simulink model "PD_funcional2018"  (R2023a)
settings: Solver=ode4  StartTime=0.0  StopTime=5  FixedStep=1e-4  RelTol=1e-3
StopFcn:
  | out = evalin('base','out');
  | animar_pendulo(out,30)
model workspace (MAT data in the model file):
  sample_time = 0.001
  sat_limit = 10
libraries: eeGeneralControl x1

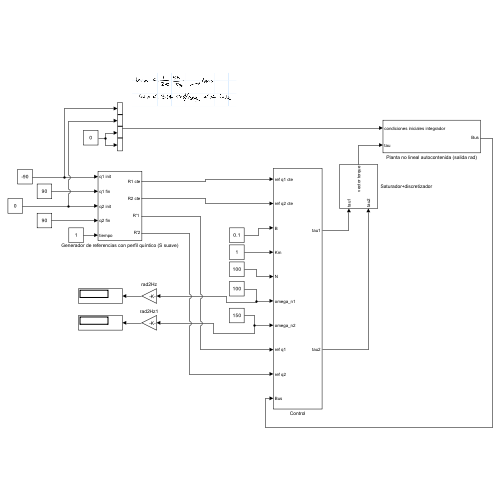
[thumbnail: Simulink's stored preview of the top-level diagram]
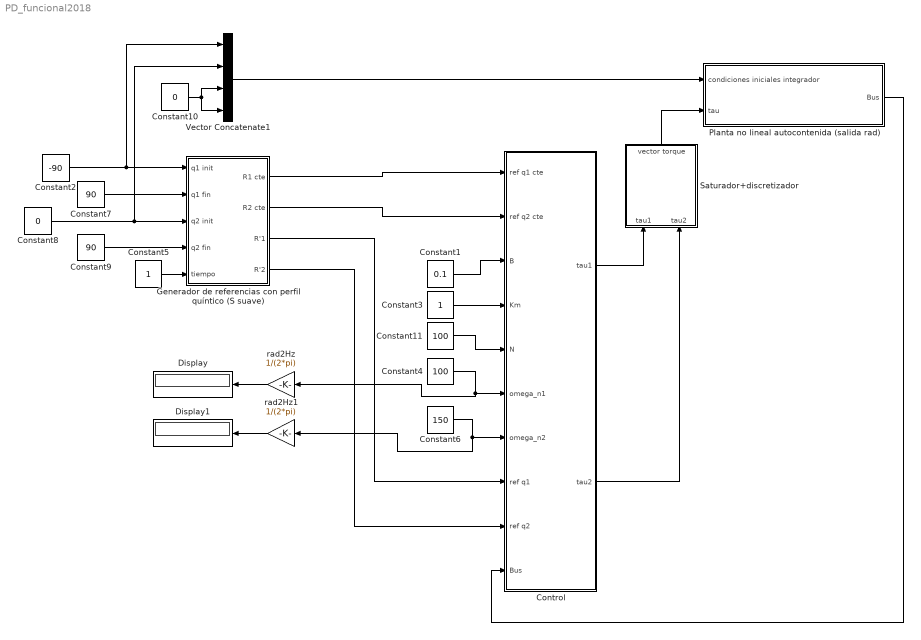
== system PD_funcional2018 ==
  Constant1 : Constant  Value=0.1
  Constant10 : Constant  Value=0
  Constant11 : Constant  Value=100
  Constant2 : Constant  Value=-90
  Constant3 : Constant
  Constant4 : Constant  Value=100
  Constant5 : Constant
  Constant6 : Constant  Value=150
  Constant7 : Constant  Value=90
  Constant8 : Constant  Value=0
  Constant9 : Constant  Value=90
  Control : Subsystem
  Display : Display
  Display1 : Display
  Generador de referencias con perfil quíntico (S suave) : Subsystem
  Planta no lineal autocontenida (salida rad) : Subsystem
  Saturador+discretizador : Subsystem
  Vector Concatenate1 : Concatenate  NumInputs=4
  rad2Hz : Gain  Gain=1/(2*pi)
  rad2Hz1 : Gain  Gain=1/(2*pi)
  wires:
  Constant2/1 -> Generador de referencias con perfil quíntico (S suave)/1(q1 init), Vector Concatenate1/1
  Constant7/1 -> Generador de referencias con perfil quíntico (S suave)/2(q1 fin)
  Constant8/1 -> Vector Concatenate1/2, Generador de referencias con perfil quíntico (S suave)/3(q2 init)
  Constant9/1 -> Generador de referencias con perfil quíntico (S suave)/4(q2 fin)
  Constant5/1 -> Generador de referencias con perfil quíntico (S suave)/5(tiempo)
  Saturador+discretizador/1(vector torque) -> Planta no lineal autocontenida (salida rad)/2(tau)
  Constant10/1 -> Vector Concatenate1/3, Vector Concatenate1/4
  Vector Concatenate1/1 -> Planta no lineal autocontenida (salida rad)/1(condiciones iniciales integrador)
  Generador de referencias con perfil quíntico (S suave)/1(R1 cte) -> Control/1(ref q1 cte)
  Generador de referencias con perfil quíntico (S suave)/2(R2 cte) -> Control/2(ref q2 cte)
  Constant1/1 -> Control/3(B)
  Constant3/1 -> Control/4(Km)
  Constant4/1 -> rad2Hz/1, Control/6(omega_n1)
  Constant6/1 -> rad2Hz1/1, Control/7(omega_n2)
  Control/1(tau1) -> Saturador+discretizador/1(tau1)
  Planta no lineal autocontenida (salida rad)/1(Bus) -> Control/10(Bus)
  Generador de referencias con perfil quíntico (S suave)/3("R'1 ") -> Control/8(ref q1)
  Generador de referencias con perfil quíntico (S suave)/4(R'2) -> Control/9(ref q2)
  rad2Hz/1 -> Display/1
  rad2Hz1/1 -> Display1/1
  Control/2(tau2) -> Saturador+discretizador/2(tau2)
  Constant11/1 -> Control/5(N)

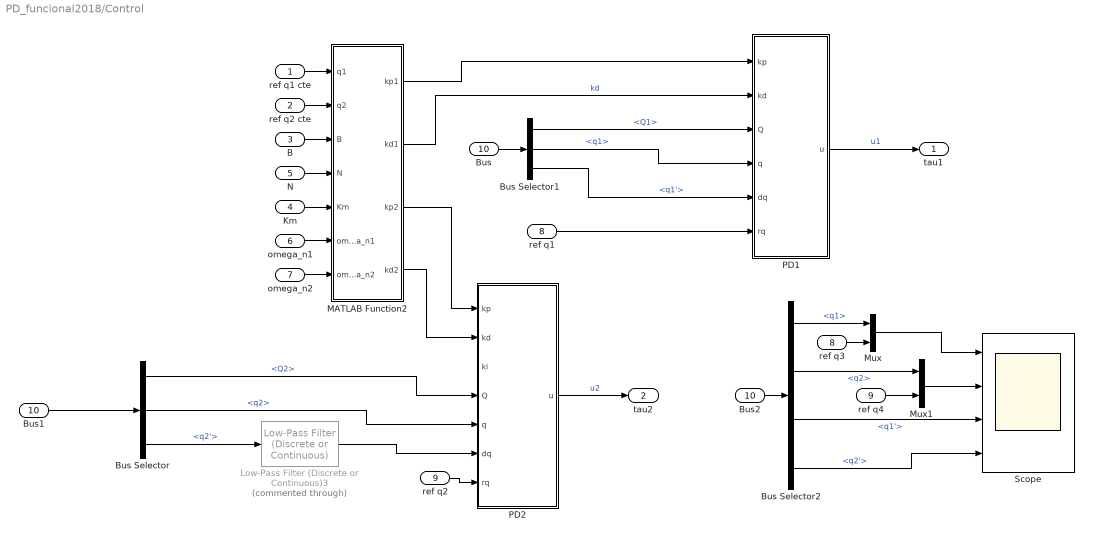
== system PD_funcional2018/Control ==
  ref q1 cte : Inport
  ref q2 cte : Inport  Port=2
  B : Inport  Port=3
  Km : Inport  Port=4
  N : Inport  Port=5
  omega_n1 : Inport  Port=6
  omega_n2 : Inport  Port=7
  ref q1 : Inport  Port=8
  ref q2 : Inport  Port=9
  Bus : Inport  Port=10
  Bus Selector : BusSelector  OutputSignals=Q2,q2,q2'
  Bus Selector1 : BusSelector  OutputSignals=Q1,q1,q1'
  Bus Selector2 : BusSelector  OutputSignals=q1,q2,q1',q2'
  Bus1 : InportShadow  Port=10
  Bus2 : InportShadow  Port=10
  Low-Pass Filter (Discrete or Continuous)3 : eeGeneralControl/Low-Pass Filter (Discrete or Continuous)  Commented=through  K=1  T=1/30  B=inf  A=-inf  init_option=Inherited from block input  x0=0  Ts=-1
  MATLAB Function2 : MATLAB Function  TreatAsAtomicUnit=on
  Mux : Mux  Inputs=2
  Mux1 : Mux  Inputs=2
  PD1 : MATLAB Function  TreatAsAtomicUnit=on
  PD2 : MATLAB Function  TreatAsAtomicUnit=on
  Scope : Scope  NumInputPorts=4
  ref q3 : InportShadow  Port=8
  ref q4 : InportShadow  Port=9
  tau1 : Outport
  tau2 : Outport  Port=2
  wires:
  ref q1 cte/1 -> MATLAB Function2/1(q1)
  ref q2 cte/1 -> MATLAB Function2/2(q2)
  B/1 -> MATLAB Function2/3(B)
  omega_n2/1 -> MATLAB Function2/7(omega_n2)
  omega_n1/1 -> MATLAB Function2/6(omega_n1)
  PD1/1(u) -> tau1/1  "u1"
  PD2/1(u) -> tau2/1  "u2"
  ref q1/1 -> PD1/6(rq)
  ref q2/1 -> PD2/7(rq)
  MATLAB Function2/1(kp1) -> PD1/1(kp)
  MATLAB Function2/3(kp2) -> PD2/1(kp)
  MATLAB Function2/2(kd1) -> PD1/2(kd)  "kd"
  MATLAB Function2/4(kd2) -> PD2/2(kd)
  Bus1/1 -> Bus Selector/1
  Bus/1 -> Bus Selector1/1
  Bus Selector1/1 -> PD1/3(Q)  "<Q1>"
  Bus Selector1/2 -> PD1/4(q)  "<q1>"
  Bus Selector1/3 -> PD1/5(dq)  "<q1'>"
  Bus Selector/1 -> PD2/4(Q)  "<Q2>"
  Bus Selector/3 -> Low-Pass Filter (Discrete or Continuous)3/1  "<q2'>"
  Mux/1 -> Scope/1
  Mux1/1 -> Scope/2
  Bus2/1 -> Bus Selector2/1
  Bus Selector2/1 -> Mux/1  "<q1>"
  Bus Selector2/2 -> Mux1/1  "<q2>"
  Bus Selector2/3 -> Scope/3  "<q1'>"
  Bus Selector2/4 -> Scope/4  "<q2'>"
  ref q3/1 -> Mux/2
  ref q4/1 -> Mux1/2
  Bus Selector/2 -> PD2/5(q)  "<q2>"
  Low-Pass Filter (Discrete or Continuous)3/1 -> PD2/6(dq)
  Km/1 -> MATLAB Function2/5(Km)
  N/1 -> MATLAB Function2/4(N)

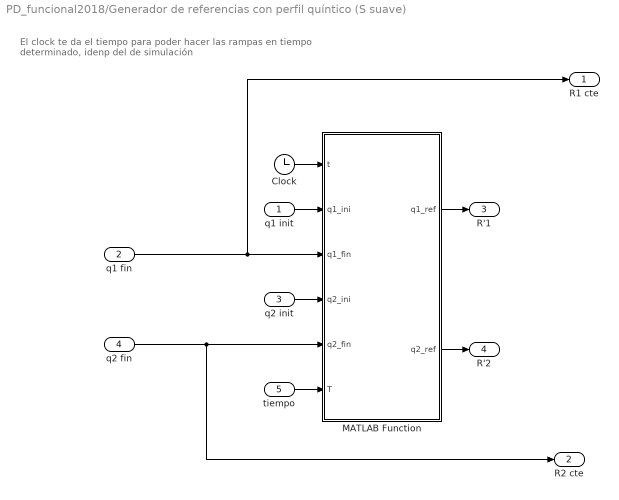
== system PD_funcional2018/Generador de referencias con perfil quíntico (S suave) ==
  note: El clock te da el tiempo para poder hacer las rampas en tiempo determinado, idenp del de simulación
  q1 init : Inport
  q1 fin : Inport  Port=2
  q2 init : Inport  Port=3
  q2 fin : Inport  Port=4
  tiempo : Inport  Port=5
  Clock : Clock
  MATLAB Function : MATLAB Function  TreatAsAtomicUnit=on
  R1 cte : Outport
  R2 cte : Outport  Port=2
  "R'1 " : Outport  Port=3
  R'2 : Outport  Port=4
  wires:
  q1 fin/1 -> R1 cte/1, MATLAB Function/3(q1_fin)
  q2 fin/1 -> R2 cte/1, MATLAB Function/5(q2_fin)
  q1 init/1 -> MATLAB Function/2(q1_ini)
  q2 init/1 -> MATLAB Function/4(q2_ini)
  MATLAB Function/1(q1_ref) -> "R'1 "/1
  MATLAB Function/2(q2_ref) -> R'2/1
  tiempo/1 -> MATLAB Function/6(T)
  Clock/1 -> MATLAB Function/1(t)

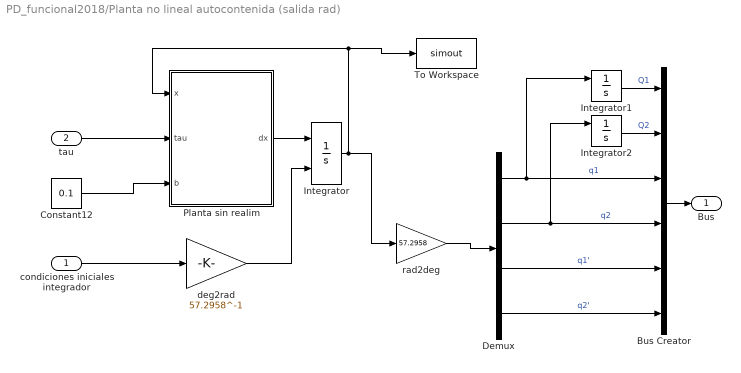
== system PD_funcional2018/Planta no lineal autocontenida (salida rad) ==
  condiciones iniciales integrador : Inport
  tau : Inport  Port=2
  Bus Creator : BusCreator  Inputs=6
  Constant12 : Constant  Value=0.1
  Demux : Demux
  Integrator : Integrator  InitialConditionSource=external
  Integrator1 : Integrator  InitialConditionSource=external
  Integrator2 : Integrator  InitialConditionSource=external
  Planta sin realim : MATLAB Function  TreatAsAtomicUnit=on
  To Workspace : ToWorkspace  VariableName=simout  SaveFormat=Structure With Time  SampleTime=-1
  deg2rad : Gain  Gain=57.2958^-1
  rad2deg : Gain  Gain=57.2958
  Bus : Outport
  wires:
  tau/1 -> Planta sin realim/2(tau)
  Constant12/1 -> Planta sin realim/3(b)
  Integrator/1 -> Planta sin realim/1(x), To Workspace/1, rad2deg/1
  condiciones iniciales integrador/1 -> deg2rad/1
  Planta sin realim/1(dx) -> Integrator/1
  deg2rad/1 -> Integrator/2
  rad2deg/1 -> Demux/1
  Demux/1 -> Integrator1/1, Bus Creator/3  "q1"
  Demux/2 -> Integrator2/1, Bus Creator/4  "q2"
  Demux/3 -> Bus Creator/5  "q1'"
  Demux/4 -> Bus Creator/6  "q2'"
  Integrator1/1 -> Bus Creator/1  "Q1"
  Integrator2/1 -> Bus Creator/2  "Q2"
  Bus Creator/1 -> Bus/1

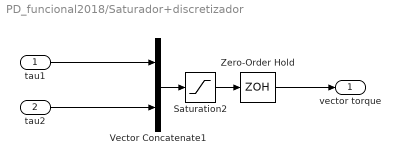
== system PD_funcional2018/Saturador+discretizador ==
  tau1 : Inport
  tau2 : Inport  Port=2
  Saturation2 : Saturate  UpperLimit=sat_limit  LowerLimit=-sat_limit
  Vector Concatenate1 : Concatenate
  Zero-Order Hold : ZeroOrderHold  SampleTime=sample_time
  vector torque : Outport
  wires:
  tau2/1 -> Vector Concatenate1/2
  tau1/1 -> Vector Concatenate1/1
  Saturation2/1 -> Zero-Order Hold/1
  Vector Concatenate1/1 -> Saturation2/1
  Zero-Order Hold/1 -> vector torque/1

== matlab function PD_funcional2018/Control/PD1 ==
function u  = PD(kp,kd,Q,q,dq,rq)
error = rq - q;
u = kp*error - kd * dq;
end

== matlab function PD_funcional2018/Planta no lineal autocontenida (salida rad)/Planta sin realim ==
function dx = modelo_estado(x, tau, b)
% MODELO_ESTADO  Bloque MATLAB Function para Simulink — formulación SS no lineal.
% Devuelve la derivada del vector de estado completo.
%
% Entradas:
%   x   = [q1; q2; dq1; dq2]  (4x1)
%   tau = [tau1; tau2]         (2x1)
%
% Salida:
%   dx  = [dq1; dq2; ddq1; ddq2]  (4x1)
%
% Conectar: un bloque Integrator vectorial (IC = x0, 4 estados)
%           con retroalimentación completa de x.

q1  = x(1);
q2  = x(2);
dq1 = x(3);
dq2 = x(4);

[ddq1, ddq2] = dinamica_fcn(q1, q2, dq1, dq2, tau(1), tau(2),b);

dx = [dq1; dq2; ddq1; ddq2];
end


function [ddq1, ddq2] = dinamica_fcn(q1, q2, dq1, dq2, tau1, tau2,b)
% DINAMICA_FCN  Bloque MATLAB Function para Simulink.
% Calcula las aceleraciones articulares del doble péndulo invertido.
% Modelo: tau = M(q)*ddq + H(q,dq) + G(q)  =>  ddq = M^-1*(tau - H - G)
%
% Notación: c1=cos(q1), s1=sin(q1), c12=cos(q1+q2), s12=sin(q1+q2), c2=cos(q2)

% --- Parámetros (hardcoded para el bloque) ---
a1    = 0.2;
a2    = 0.2;
m1    = 1.5;
m2    = 1.0;
Ig1zz = 1e-3;
Ig2zz = 1e-4;
xg1   = -a1/2;   % = -0.1
yg1   = 0;
xg2   = -a2/2;   % = -0.1
yg2   = 0;
grav  = 9.81;

% --- Trigonometría ---
c1  = cos(q1);
s1  = sin(q1);
c2  = cos(q2);
s2  = sin(q2);
c12 = cos(q1 + q2);
s12 = sin(q1 + q2);

% --- Matriz de inercia M (ec. 27-30 de la memoria) ---
% I0izz = Igizz + (xgi^2 + ygi^2)*mi  [Steiner, para la terna del eslabón]
I01zz = Ig1zz + (xg1^2 + yg1^2)*m1;   % = 0.016 Kg·m²
I02zz = Ig2zz + (xg2^2 + yg2^2)*m2;   % = 0.0101 Kg·m²  (aprox, yg2=0)

m22 = I02zz + 2*a2*xg2*m2 + a2^2*m2;
m12 = m22 + a1*((a2 + xg2)*c2 - yg2*s2)*m2;
m11 = I01zz + 2*a1*xg1*m1 + a1^2*(m1 + m2) + 2*m12 - m22;

M = [m11, m12; m12, m22];

% --- Vector H — Coriolis y centrífugo (ec. 33) ---
dm12_dq2 = -a1*((a2 + xg2)*s2 + yg2*c2)*m2;

H1 = dm12_dq2 * (2*dq1*dq2 + dq2^2);
H2 = -dm12_dq2 * dq1^2;

H = [H1; H2];

% --- Vector G — gravedad (ec. 36, 40) ---
% g^0 = [0, -9.81, 0]^t  (montado en la pared, gravedad en -Y de frame 0)
g2 = m2*grav*((xg2 + a2)*c12 - yg2*s12);
g1 = m1*grav*((xg1 + a1)*c1 - yg1*s1) + m2*grav*a1*c1 + g2;

G = [g1; g2];

B = [dq1; dq2] * b; % fricción simplificada

% --- Ecuación de movimiento ---
tau = [tau1; tau2];
ddq = M \ (tau - H - G - B); % no está dividiendo, esta resolviendo con división de M a izquierda
% B es fricción 

ddq1 = ddq(1);
ddq2 = ddq(2);
end

== matlab function PD_funcional2018/Control/MATLAB Function2 ==
function [kp1,kd1,kp2,kd2] = coefs_PD(q1,q2,B,N,Km,omega_n1,omega_n2)
%e error
[Jef1,Jef2] = Matriz_M_eq(q1,q2);

kp1 = (omega_n1^2)*Jef1 / (N*Km);
kd1 = (2 * sqrt(N*Km*kp1*Jef1)- B)/(N*Km); 

kp2 = (omega_n2^2)*Jef2 / (N*Km);
kd2 = (2 * sqrt(N*Km*kp2*Jef2)- B)/(N*Km); 

end

function [m11,m22] = Matriz_M_eq(q1, q2)
% DINAMICA_FCN  Bloque MATLAB Function para Simulink.
% Calcula las aceleraciones articulares del doble péndulo invertido.
% Modelo: tau = M(q)*ddq + H(q,dq) + G(q)  =>  ddq = M^-1*(tau - H - G)
%
% Notación: c1=cos(q1), s1=sin(q1), c12=cos(q1+q2), s12=sin(q1+q2), c2=cos(q2)

% --- Parámetros (hardcoded para el bloque) ---
a1    = 0.2;
a2    = 0.2;
m1    = 1.5;
m2    = 1.0;
Ig1zz = 1e-3;
Ig2zz = 1e-4;
xg1   = -a1/2;   % = -0.1
yg1   = 0;
xg2   = -a2/2;   % = -0.1
yg2   = 0;
grav  = 9.81;

q1 = deg2rad(q1);
q2 = deg2rad(q2);

% --- Trigonometría ---
c1  = cos(q1);
s1  = sin(q1);
c2  = cos(q2);
s2  = sin(q2);
c12 = cos(q1 + q2);
s12 = sin(q1 + q2);

% --- Matriz de inercia M (ec. 27-30 de la memoria) ---
% I0izz = Igizz + (xgi^2 + ygi^2)*mi  [Steiner, para la terna del eslabón]
I01zz = Ig1zz + (xg1^2 + yg1^2)*m1;   % = 0.016 Kg·m²
I02zz = Ig2zz + (xg2^2 + yg2^2)*m2;   % = 0.0101 Kg·m²  (aprox, yg2=0)

m22 = I02zz + 2*a2*xg2*m2 + a2^2*m2;
m12 = m22 + a1*((a2 + xg2)*c2 - yg2*s2)*m2;
m11 = I01zz + 2*a1*xg1*m1 + a1^2*(m1 + m2) + 2*m12 - m22;

M = [m11, m12; m12, m22];

m11=m11;
m12=m12;
m21=m12;
m22=m22;
end

== matlab function PD_funcional2018/Control/PD2 ==
function u  = PD(kp,kd,ki,Q,q,dq,rq)
error = rq - q;
u = kp*error - kd * dq;
end

== matlab function PD_funcional2018/Generador de referencias con perfil quíntico (S suave)/MATLAB Function ==
function [q1_ref, q2_ref] = trayectoria_perfil_quitico(t,q1_ini, q1_fin,q2_ini, q2_fin,T)

% TRAYECTORIA_LINEAL
% Genera una interpolación lineal entre dos posiciones articulares.
%
% Entradas:
%   t        -> tiempo actual
%   q1_ini   -> ángulo inicial q1 [deg]
%   q1_fin   -> ángulo final q1 [deg]
%   q2_ini   -> ángulo inicial q2 [deg]
%   q2_fin   -> ángulo final q2 [deg]
%   T        -> duración total del movimiento [s]
%
% Salidas:
%   q1_ref   -> referencia q1 [deg]
%   q2_ref   -> referencia q2 [deg]

if t <= 0

    s = 0;

elseif t >= T

    s = 1;

else

    s = t/T;

end

h = 10*s^3 - 15*s^4 + 6*s^5;

q1_ref = q1_ini + (q1_fin - q1_ini)*h;
q2_ref = q2_ini + (q2_fin - q2_ini)*h;

end
